simulink model "sk_QR_Unbalanced"  (Simulink 8.4)
settings: Solver=ode45  StartTime=0.0  StopTime=11  MaxStep=1e-3  RelTol=1e-3
settings Model: Creator=Isa  LastModifiedBy=etsi  ExtModeTrigMode=oneshot  ExtModeArmWhenConnect=off
settings DataIOCC: LimitDataPoints=off
settings OptimizationCC: BlockReduction=off  BooleanDataType=off  InitFltsAndDblsToZero=on
settings DebuggingCC: SaveWithParameterizedLinksMsg=none  SignalResolutionControl=TryResolveAllWithWarning  SolverPrmCheckMsg=none  MultiTaskDSMMsg=warning  MultiTaskCondExecSysMsg=none
settings HardwareCC: TargetUnknown=on
settings RTWCC: IncludeERTFirstTime=on
settings GRTTargetCC: TargetFcnLib=ansi_tfl_tmw.mat

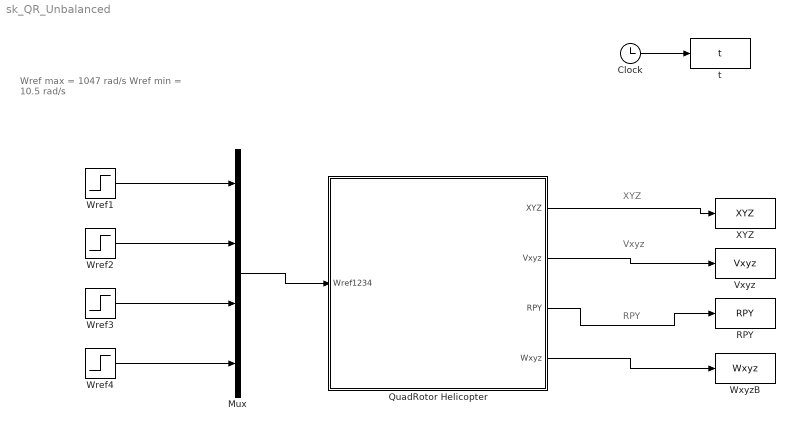
== system sk_QR_Unbalanced ==
  note: XYZ
  note: Vxyz
  note: RPY
  note: Wref max = 1047 rad/s
      | Wref min = 10.5 rad/s
  Clock : Clock
  Mux : Mux
  QuadRotor Helicopter : Subsystem  mask(Balanced Quadrotor Helicopter){X_ini=0, Y_ini=0, Z_ini=0}
      mask prompts: X_ini "X inicial (m)"; Y_ini "Y inicial (m)"; Z_ini "Z inicial (m)"
      mask help: Inputs: speed reference for each rotor.
      mask Display:
      | image(imread('QR.JPG'));
      | port_label('output', 1, 'XYZ');
      | port_label('output', 2, 'Vxyz');
      | port_label('output', 3, 'RPY');
      | port_label('output', 4, 'Wxyz');
      | port_label('input', 1, 'Wmref')
  RPY : ToWorkspace  VariableName=RPY  SampleTime=-1
  Vxyz : ToWorkspace  VariableName=Vxyz  SampleTime=-1
  Wref1 : Step  Before=760.44  After=760.44*1.02  SampleTime=0
  Wref2 : Step  Before=760.44  After=760.44*0.98  SampleTime=0
  Wref3 : Step  Before=760.44  After=760.44*1.02  SampleTime=0
  Wref4 : Step  Before=760.44  After=760.44  SampleTime=0
  WxyzB : ToWorkspace  VariableName=Wxyz  SampleTime=-1
  XYZ : ToWorkspace  VariableName=XYZ  SampleTime=-1
  t : ToWorkspace  VariableName=t  SampleTime=-1
  wires:
  Clock/1 -> t/1
  QuadRotor Helicopter/1(XYZ) -> XYZ/1
  QuadRotor Helicopter/3(RPY) -> RPY/1
  QuadRotor Helicopter/2(Vxyz) -> Vxyz/1
  QuadRotor Helicopter/4(Wxyz) -> WxyzB/1
  Wref1/1 -> Mux/1
  Wref2/1 -> Mux/2
  Wref3/1 -> Mux/3
  Wref4/1 -> Mux/4
  Mux/1 -> QuadRotor Helicopter/1(Wref1234)

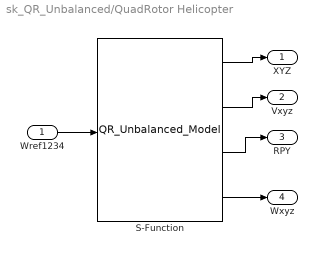
== system sk_QR_Unbalanced/QuadRotor Helicopter ==
  Wref1234 : Inport
  S-Function : S-Function  FunctionName=QR_Unbalanced_Model  Parameters=[X_ini, Y_ini, Z_ini]  EnableBusSupport=off
  XYZ : Outport
  Vxyz : Outport  Port=2
  RPY : Outport  Port=3
  Wxyz : Outport  Port=4
  wires:
  Wref1234/1 -> S-Function/1
  S-Function/1 -> XYZ/1
  S-Function/2 -> Vxyz/1
  S-Function/3 -> RPY/1
  S-Function/4 -> Wxyz/1
